simulink model "Absolute_Block_Testing"  (R2021a)
settings: Solver=VariableStepAuto  StartTime=0.0  StopTime=0.35  RelTol=1e-3
undefined symbols (not defined in the file): lambda2
libraries: dspsigops x4, dspquant2 x4
(part 1 of 2)
settings Model: Creator=hp  LastModifiedBy=hp

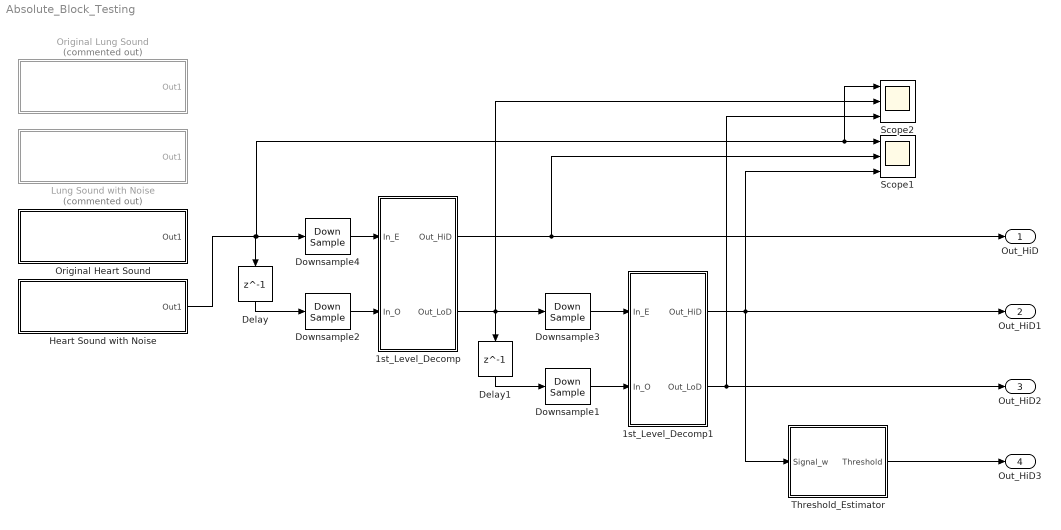
== system Absolute_Block_Testing ==
  1st_Level_Decomp : Subsystem
  1st_Level_Decomp1 : Subsystem
  Delay : Delay  DelayLength=1  SampleTime=1/44100
  Delay1 : Delay  DelayLength=1  SampleTime=1/44100
  Downsample{1..4} (4 alike) : DownSample  N=20  RateOptions=Allow multirate processing
  Heart Sound with Noise : Subsystem
  Lung Sound with Noise : Subsystem  Commented=on
  Original Heart Sound : Subsystem
  Original Lung Sound : Subsystem  Commented=on
  Scope1 : Scope  NumInputPorts=3
  Scope2 : Scope  NumInputPorts=3
  Threshold_Estimator : Subsystem
  Out_HiD : Outport  OutDataTypeStr=fixdt(1,16,12)  SampleTime=1/44100  VectorParamsAs1DForOutWhenUnconnected=off
  Out_HiD1 : Outport  Port=2  OutDataTypeStr=fixdt(1,16,12)  SampleTime=1/44100  VectorParamsAs1DForOutWhenUnconnected=off
  Out_HiD2 : Outport  Port=3  OutDataTypeStr=fixdt(1,16,12)  SampleTime=1/44100  VectorParamsAs1DForOutWhenUnconnected=off
  Out_HiD3 : Outport  Port=4  OutDataTypeStr=fixdt(1,16,12)  SampleTime=1/44100  VectorParamsAs1DForOutWhenUnconnected=off
  wires:
  Delay/1 -> Downsample2/1
  Downsample2/1 -> 1st_Level_Decomp/2(In_O)
  Downsample4/1 -> 1st_Level_Decomp/1(In_E)
  Downsample3/1 -> 1st_Level_Decomp1/1(In_E)
  Delay1/1 -> Downsample1/1
  1st_Level_Decomp/2(Out_LoD) -> Scope2/2, Delay1/1, Downsample3/1
  Downsample1/1 -> 1st_Level_Decomp1/2(In_O)
  1st_Level_Decomp1/1(Out_HiD) -> Scope1/3, Out_HiD1/1, Threshold_Estimator/1(Signal_w)
  1st_Level_Decomp/1(Out_HiD) -> Scope1/2, Out_HiD/1
  1st_Level_Decomp1/2(Out_LoD) -> Scope2/3, Out_HiD2/1
  Threshold_Estimator/1(Threshold) -> Out_HiD3/1
  Heart Sound with Noise/1(Out1) -> Delay/1, Scope1/1, Scope2/1, Downsample4/1

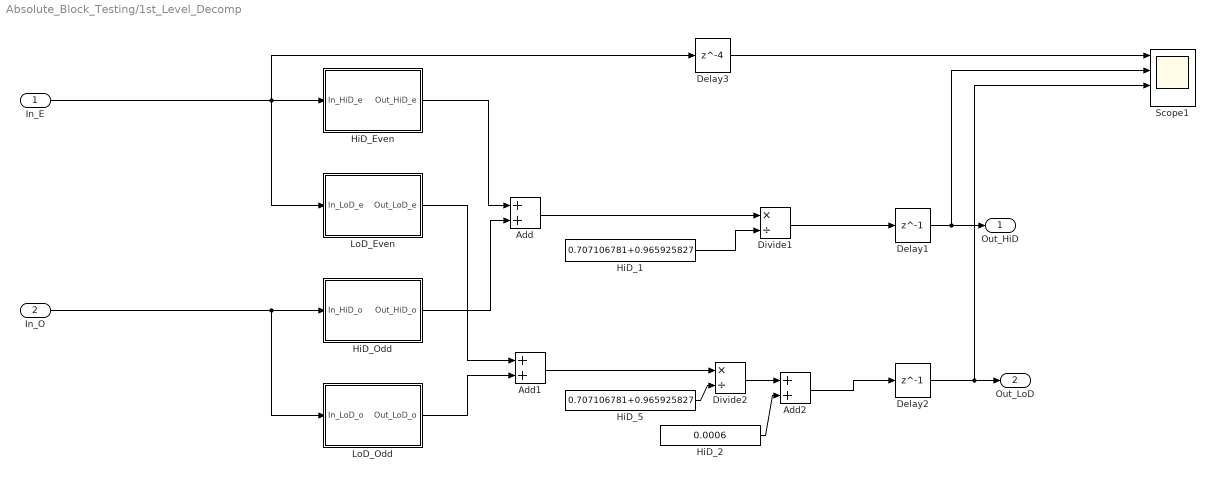
== system Absolute_Block_Testing/1st_Level_Decomp ==
  In_E : Inport  OutDataTypeStr=fixdt(1,16,12)  SampleTime=0.000022675736
  In_O : Inport  Port=2  OutDataTypeStr=fixdt(1,16,12)  SampleTime=0.000022675736
  Add : Sum  AccumDataTypeStr=fixdt(1,16,12)  OutDataTypeStr=fixdt(1,16,12)  LockScale=on
  Add1 : Sum  AccumDataTypeStr=fixdt(1,16,12)  OutDataTypeStr=fixdt(1,16,12)  LockScale=on
  Add2 : Sum  AccumDataTypeStr=fixdt(1,16,12)  OutDataTypeStr=fixdt(1,16,12)  LockScale=on
  Delay1 : Delay  DelayLength=1  SampleTime=0.000022675736
  Delay2 : Delay  DelayLength=1  SampleTime=0.000022675736
  Delay3 : Delay  DelayLength=4  SampleTime=0.000022675736
  Divide1 : Product  Inputs=*/  OutDataTypeStr=fixdt(1,16,12)
  Divide2 : Product  Inputs=*/  OutDataTypeStr=fixdt(1,16,12)
  HiD_1 : Constant  Value=0.707106781+0.965925827  OutDataTypeStr=fixdt(1,16,12)  SampleTime=1/44100
  HiD_2 : Constant  Value=0.0006  OutDataTypeStr=fixdt(1,16,12)  SampleTime=1/44100
  HiD_5 : Constant  Value=0.707106781+0.965925827  OutDataTypeStr=fixdt(1,16,12)  SampleTime=1/44100
  HiD_Even : Subsystem
  HiD_Odd : Subsystem
  LoD_Even : Subsystem
  LoD_Odd : Subsystem
  Scope1 : Scope  NumInputPorts=4
  Out_HiD : Outport  OutDataTypeStr=fixdt(1,16,12)  SampleTime=0.000022675736
  Out_LoD : Outport  Port=2  OutDataTypeStr=fixdt(1,16,12)  SampleTime=0.000022675736
  wires:
  HiD_Even/1(Out_HiD_e) -> Add/1
  HiD_Odd/1(Out_HiD_o) -> Add/2
  LoD_Even/1(Out_LoD_e) -> Add1/1
  Delay1/1 -> Scope1/2, Out_HiD/1
  Delay2/1 -> Scope1/3, Out_LoD/1
  In_E/1 -> LoD_Even/1(In_LoD_e), Delay3/1, HiD_Even/1(In_HiD_e)
  In_O/1 -> HiD_Odd/1(In_HiD_o), LoD_Odd/1(In_LoD_o)
  Add/1 -> Divide1/1
  Add1/1 -> Divide2/1
  LoD_Odd/1(Out_LoD_o) -> Add1/2
  HiD_5/1 -> Divide2/2
  HiD_1/1 -> Divide1/2
  Delay3/1 -> Scope1/1
  Divide2/1 -> Add2/1
  HiD_2/1 -> Add2/2
  Add2/1 -> Delay2/1
  Divide1/1 -> Delay1/1

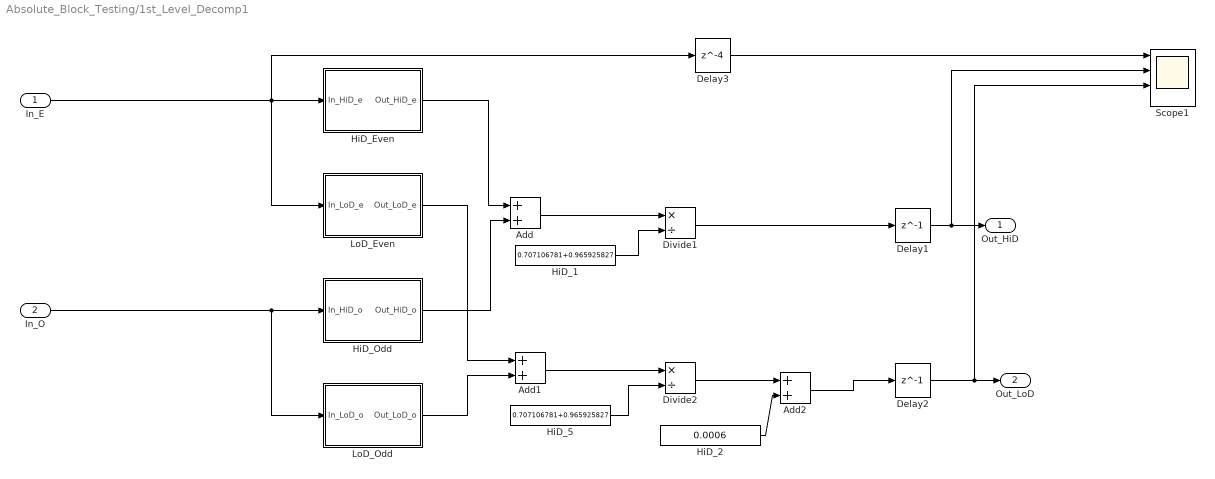
== system Absolute_Block_Testing/1st_Level_Decomp1 ==
  In_E : Inport  OutDataTypeStr=fixdt(1,16,12)  SampleTime=0.000022675736
  In_O : Inport  Port=2  OutDataTypeStr=fixdt(1,16,12)  SampleTime=0.000022675736
  Add : Sum  AccumDataTypeStr=fixdt(1,16,12)  OutDataTypeStr=fixdt(1,16,12)  LockScale=on
  Add1 : Sum  AccumDataTypeStr=fixdt(1,16,12)  OutDataTypeStr=fixdt(1,16,12)  LockScale=on
  Add2 : Sum  AccumDataTypeStr=fixdt(1,16,12)  OutDataTypeStr=fixdt(1,16,12)  LockScale=on
  Delay1 : Delay  DelayLength=1  SampleTime=0.000022675736
  Delay2 : Delay  DelayLength=1  SampleTime=0.000022675736
  Delay3 : Delay  DelayLength=4  SampleTime=0.000022675736
  Divide1 : Product  Inputs=*/  OutDataTypeStr=fixdt(1,16,12)
  Divide2 : Product  Inputs=*/  OutDataTypeStr=fixdt(1,16,12)
  HiD_1 : Constant  Value=0.707106781+0.965925827  OutDataTypeStr=fixdt(1,16,12)  SampleTime=1/44100
  HiD_2 : Constant  Value=0.0006  OutDataTypeStr=fixdt(1,16,12)  SampleTime=1/44100
  HiD_5 : Constant  Value=0.707106781+0.965925827  OutDataTypeStr=fixdt(1,16,12)  SampleTime=1/44100
  HiD_Even : Subsystem
  HiD_Odd : Subsystem
  LoD_Even : Subsystem
  LoD_Odd : Subsystem
  Scope1 : Scope  NumInputPorts=4
  Out_HiD : Outport  OutDataTypeStr=fixdt(1,16,12)  SampleTime=0.000022675736
  Out_LoD : Outport  Port=2  OutDataTypeStr=fixdt(1,16,12)  SampleTime=0.000022675736
  wires:
  HiD_Even/1(Out_HiD_e) -> Add/1
  HiD_Odd/1(Out_HiD_o) -> Add/2
  LoD_Even/1(Out_LoD_e) -> Add1/1
  Delay1/1 -> Scope1/2, Out_HiD/1
  Delay2/1 -> Scope1/3, Out_LoD/1
  In_E/1 -> LoD_Even/1(In_LoD_e), Delay3/1, HiD_Even/1(In_HiD_e)
  In_O/1 -> HiD_Odd/1(In_HiD_o), LoD_Odd/1(In_LoD_o)
  Add/1 -> Divide1/1
  Add1/1 -> Divide2/1
  LoD_Odd/1(Out_LoD_o) -> Add1/2
  HiD_5/1 -> Divide2/2
  HiD_1/1 -> Divide1/2
  Delay3/1 -> Scope1/1
  Divide2/1 -> Add2/1
  HiD_2/1 -> Add2/2
  Add2/1 -> Delay2/1
  Divide1/1 -> Delay1/1

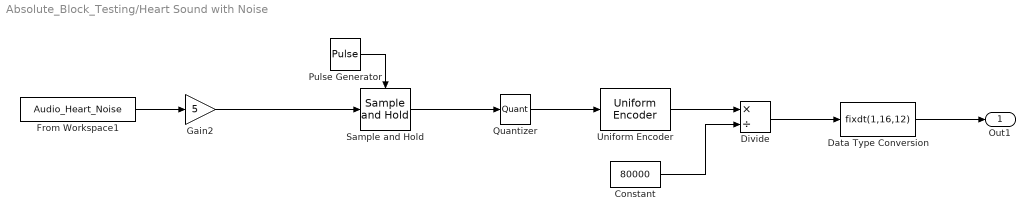
== system Absolute_Block_Testing/Heart Sound with Noise ==
  Constant : Constant  Value=80000
  Data Type Conversion : DataTypeConversion  OutDataTypeStr=fixdt(1,16,12)
  Divide : Product  Inputs=*/
  From Workspace1 : FromWorkspace  VariableName=Audio_Heart_Noise  OutDataTypeStr=double
  Gain2 : Gain  Gain=5
  Pulse Generator : DiscretePulseGenerator  PulseType=Time based  Period=0.00022675736  PulseWidth=50
  Quantizer : Quantizer  QuantizationInterval=0.1
  Sample and Hold : dspsigops/Sample and Hold  trig=Rising edge  initCond=0  latchinput=off
  Uniform Encoder : dspquant2/Uniform Encoder  peak=2  bits=8  otype=Unsigned integer
  Out1 : Outport  OutDataTypeStr=fixdt(1,16,12)  SampleTime=1/44100
  wires:
  Sample and Hold/1 -> Quantizer/1
  Uniform Encoder/1 -> Divide/1
  Divide/1 -> Data Type Conversion/1
  Quantizer/1 -> Uniform Encoder/1
  Constant/1 -> Divide/2
  From Workspace1/1 -> Gain2/1
  Pulse Generator/1 -> Sample and Hold/Trigger
  Gain2/1 -> Sample and Hold/1
  Data Type Conversion/1 -> Out1/1

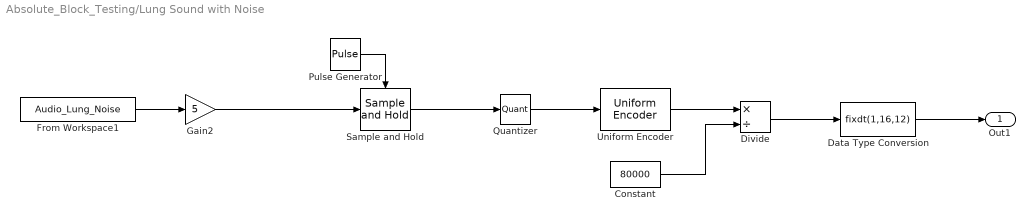
== system Absolute_Block_Testing/Lung Sound with Noise ==
  Constant : Constant  Value=80000
  Data Type Conversion : DataTypeConversion  OutDataTypeStr=fixdt(1,16,12)
  Divide : Product  Inputs=*/
  From Workspace1 : FromWorkspace  VariableName=Audio_Lung_Noise  OutDataTypeStr=double
  Gain2 : Gain  Gain=5
  Pulse Generator : DiscretePulseGenerator  PulseType=Time based  Period=0.00022675736  PulseWidth=50
  Quantizer : Quantizer  QuantizationInterval=0.1
  Sample and Hold : dspsigops/Sample and Hold  trig=Rising edge  initCond=0  latchinput=off
  Uniform Encoder : dspquant2/Uniform Encoder  peak=2  bits=8  otype=Unsigned integer
  Out1 : Outport  OutDataTypeStr=fixdt(1,16,12)  SampleTime=1/44100
  wires:
  Sample and Hold/1 -> Quantizer/1
  Uniform Encoder/1 -> Divide/1
  Divide/1 -> Data Type Conversion/1
  Quantizer/1 -> Uniform Encoder/1
  Constant/1 -> Divide/2
  From Workspace1/1 -> Gain2/1
  Pulse Generator/1 -> Sample and Hold/Trigger
  Gain2/1 -> Sample and Hold/1
  Data Type Conversion/1 -> Out1/1

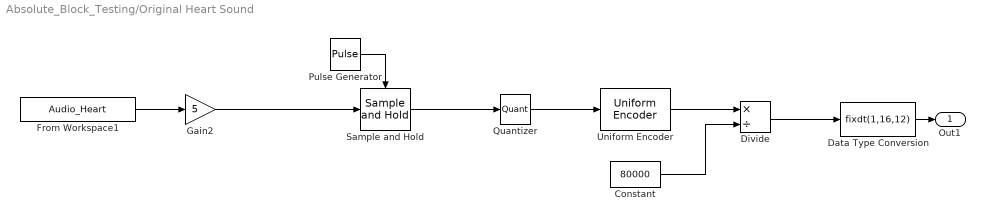
== system Absolute_Block_Testing/Original Heart Sound ==
  Constant : Constant  Value=80000
  Data Type Conversion : DataTypeConversion  OutDataTypeStr=fixdt(1,16,12)
  Divide : Product  Inputs=*/
  From Workspace1 : FromWorkspace  VariableName=Audio_Heart  OutDataTypeStr=double
  Gain2 : Gain  Gain=5
  Pulse Generator : DiscretePulseGenerator  PulseType=Time based  Period=0.00022675736  PulseWidth=50
  Quantizer : Quantizer  QuantizationInterval=0.1
  Sample and Hold : dspsigops/Sample and Hold  trig=Rising edge  initCond=0  latchinput=off
  Uniform Encoder : dspquant2/Uniform Encoder  peak=2  bits=8  otype=Unsigned integer
  Out1 : Outport  OutDataTypeStr=fixdt(1,16,12)  SampleTime=1/44100
  wires:
  Sample and Hold/1 -> Quantizer/1
  Uniform Encoder/1 -> Divide/1
  Divide/1 -> Data Type Conversion/1
  Quantizer/1 -> Uniform Encoder/1
  Constant/1 -> Divide/2
  From Workspace1/1 -> Gain2/1
  Pulse Generator/1 -> Sample and Hold/Trigger
  Gain2/1 -> Sample and Hold/1
  Data Type Conversion/1 -> Out1/1

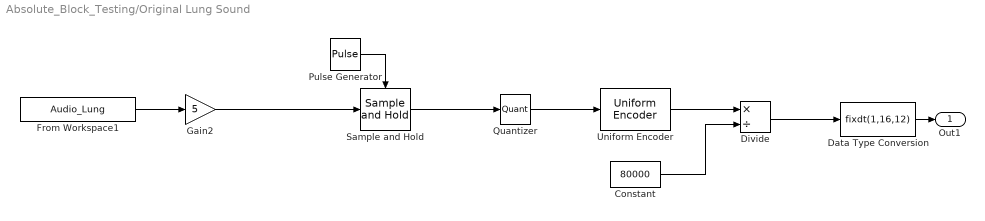
== system Absolute_Block_Testing/Original Lung Sound ==
  Constant : Constant  Value=80000
  Data Type Conversion : DataTypeConversion  OutDataTypeStr=fixdt(1,16,12)
  Divide : Product  Inputs=*/
  From Workspace1 : FromWorkspace  VariableName=Audio_Lung  OutDataTypeStr=double
  Gain2 : Gain  Gain=5
  Pulse Generator : DiscretePulseGenerator  PulseType=Time based  Period=0.00022675736  PulseWidth=50
  Quantizer : Quantizer  QuantizationInterval=0.1
  Sample and Hold : dspsigops/Sample and Hold  trig=Rising edge  initCond=0  latchinput=off
  Uniform Encoder : dspquant2/Uniform Encoder  peak=2  bits=8  otype=Unsigned integer
  Out1 : Outport  OutDataTypeStr=fixdt(1,16,12)
  wires:
  Sample and Hold/1 -> Quantizer/1
  Uniform Encoder/1 -> Divide/1
  Divide/1 -> Data Type Conversion/1
  Quantizer/1 -> Uniform Encoder/1
  Constant/1 -> Divide/2
  From Workspace1/1 -> Gain2/1
  Pulse Generator/1 -> Sample and Hold/Trigger
  Gain2/1 -> Sample and Hold/1
  Data Type Conversion/1 -> Out1/1

== system Absolute_Block_Testing/Threshold_Estimator ==
  Signal_w : Inport  OutDataTypeStr=fixdt(1,16,12)  SampleTime=0.000022675736
  Absolute Signal : Scope
  Absolute_Value1 : Subsystem
  Detailed SIgnal : Scope
  Length : Constant  Value=lambda2  OutDataTypeStr=fixdt(1,16,12)  SampleTime=0.000022675736
  Median2 : Subsystem
  Multiply : Product  OutDataTypeStr=fixdt(1,16,12)  LockScale=on
  Scope3 : Scope  NumInputPorts=2
  Threshold : Outport  OutDataTypeStr=fixdt(1,16,12)  SampleTime=0.000022675736  VectorParamsAs1DForOutWhenUnconnected=off
  wires:
  Length/1 -> Multiply/2
  Median2/1(Median) -> Multiply/1
  Absolute_Value1/1(Out_Abs) -> Absolute Signal/1, Scope3/2, Median2/1(Signal_w3)
  Signal_w/1 -> Detailed SIgnal/1, Scope3/1, Absolute_Value1/1(Signal_w4)
  Multiply/1 -> Threshold/1

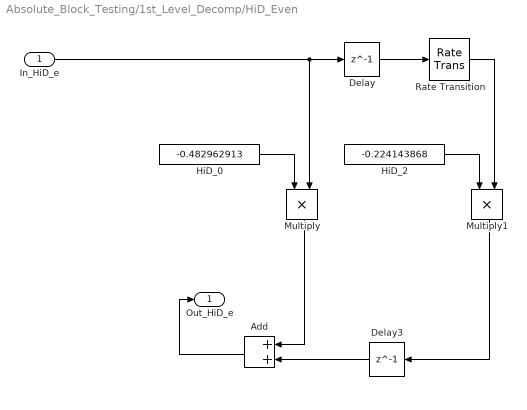
== system Absolute_Block_Testing/1st_Level_Decomp/HiD_Even ==
  In_HiD_e : Inport  OutDataTypeStr=fixdt(1,16,12)  SampleTime=0.000022675736
  Add : Sum  AccumDataTypeStr=fixdt(1,16,12)  OutDataTypeStr=fixdt(1,16,12)  LockScale=on
  Delay : Delay  DelayLength=1  SampleTime=0.000022675736
  Delay3 : Delay  DelayLength=1  SampleTime=0.000022675736
  HiD_0 : Constant  Value=-0.482962913  OutDataTypeStr=fixdt(1,16,12)  SampleTime=0.000022675736
  HiD_2 : Constant  Value=-0.224143868  OutDataTypeStr=fixdt(1,16,12)  SampleTime=0.000022675736
  Multiply : Product  OutDataTypeStr=fixdt(1,16,12)  LockScale=on
  Multiply1 : Product  OutDataTypeStr=fixdt(1,16,12)  LockScale=on
  Rate Transition : RateTransition  OutPortSampleTime=0.000022675736
  Out_HiD_e : Outport  OutDataTypeStr=fixdt(1,16,12)  SampleTime=0.000022675736  VectorParamsAs1DForOutWhenUnconnected=off
  wires:
  Delay/1 -> Rate Transition/1
  Delay3/1 -> Add/2
  Multiply1/1 -> Delay3/1
  Multiply/1 -> Add/1
  HiD_0/1 -> Multiply/1
  HiD_2/1 -> Multiply1/1
  Add/1 -> Out_HiD_e/1
  In_HiD_e/1 -> Multiply/2, Delay/1
  Rate Transition/1 -> Multiply1/2

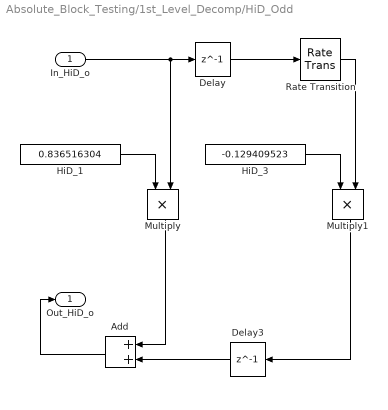
== system Absolute_Block_Testing/1st_Level_Decomp/HiD_Odd ==
  In_HiD_o : Inport  OutDataTypeStr=fixdt(1,16,12)  SampleTime=0.000022675736
  Add : Sum  AccumDataTypeStr=fixdt(1,16,12)  OutDataTypeStr=fixdt(1,16,12)  LockScale=on
  Delay : Delay  DelayLength=1  SampleTime=0.000022675736
  Delay3 : Delay  DelayLength=1  SampleTime=0.000022675736
  HiD_1 : Constant  Value=0.836516304  OutDataTypeStr=fixdt(1,16,12)  SampleTime=0
  HiD_3 : Constant  Value=-0.129409523  OutDataTypeStr=fixdt(1,16,12)  SampleTime=0
  Multiply : Product  OutDataTypeStr=fixdt(1,16,12)  LockScale=on
  Multiply1 : Product  OutDataTypeStr=fixdt(1,16,12)  LockScale=on
  Rate Transition : RateTransition  OutPortSampleTime=0.000022675736
  Out_HiD_o : Outport  OutDataTypeStr=fixdt(1,16,12)  SampleTime=0.000022675736  VectorParamsAs1DForOutWhenUnconnected=off
  wires:
  Delay/1 -> Rate Transition/1
  Delay3/1 -> Add/2
  Multiply1/1 -> Delay3/1
  Multiply/1 -> Add/1
  HiD_1/1 -> Multiply/1
  HiD_3/1 -> Multiply1/1
  Add/1 -> Out_HiD_o/1
  In_HiD_o/1 -> Delay/1, Multiply/2
  Rate Transition/1 -> Multiply1/2

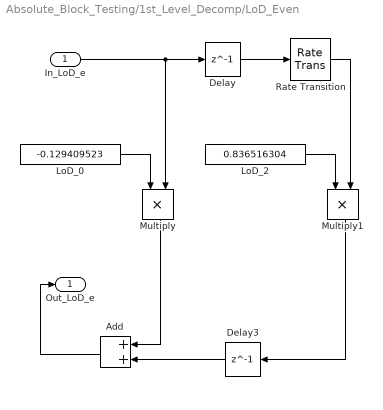
== system Absolute_Block_Testing/1st_Level_Decomp/LoD_Even ==
  In_LoD_e : Inport  OutDataTypeStr=fixdt(1,16,12)  SampleTime=0.000022675736
  Add : Sum  AccumDataTypeStr=fixdt(1,16,12)  OutDataTypeStr=fixdt(1,16,12)  LockScale=on
  Delay : Delay  DelayLength=1  SampleTime=0.000022675736
  Delay3 : Delay  DelayLength=1  SampleTime=0.000022675736
  LoD_0 : Constant  Value=-0.129409523  OutDataTypeStr=fixdt(1,16,12)  SampleTime=0
  LoD_2 : Constant  Value=0.836516304  OutDataTypeStr=fixdt(1,16,12)  SampleTime=0
  Multiply : Product  OutDataTypeStr=fixdt(1,16,12)  LockScale=on
  Multiply1 : Product  OutDataTypeStr=fixdt(1,16,12)  LockScale=on
  Rate Transition : RateTransition  OutPortSampleTime=0.000022675736
  Out_LoD_e : Outport  OutDataTypeStr=fixdt(1,16,12)  SampleTime=0.000022675736  VectorParamsAs1DForOutWhenUnconnected=off
  wires:
  Delay/1 -> Rate Transition/1
  Delay3/1 -> Add/2
  Multiply1/1 -> Delay3/1
  Multiply/1 -> Add/1
  LoD_0/1 -> Multiply/1
  LoD_2/1 -> Multiply1/1
  Add/1 -> Out_LoD_e/1
  In_LoD_e/1 -> Delay/1, Multiply/2
  Rate Transition/1 -> Multiply1/2

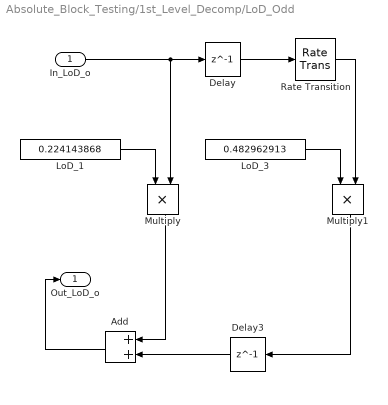
== system Absolute_Block_Testing/1st_Level_Decomp/LoD_Odd ==
  In_LoD_o : Inport  OutDataTypeStr=fixdt(1,16,12)  SampleTime=0.000022675736
  Add : Sum  AccumDataTypeStr=fixdt(1,16,12)  OutDataTypeStr=fixdt(1,16,12)  LockScale=on
  Delay : Delay  DelayLength=1  SampleTime=0.000022675736
  Delay3 : Delay  DelayLength=1  SampleTime=0.000022675736
  LoD_1 : Constant  Value=0.224143868  OutDataTypeStr=fixdt(1,16,12)  SampleTime=0
  LoD_3 : Constant  Value=0.482962913  OutDataTypeStr=fixdt(1,16,12)  SampleTime=0
  Multiply : Product  OutDataTypeStr=fixdt(1,16,12)  LockScale=on
  Multiply1 : Product  OutDataTypeStr=fixdt(1,16,12)  LockScale=on
  Rate Transition : RateTransition  OutPortSampleTime=0.000022675736
  Out_LoD_o : Outport  OutDataTypeStr=fixdt(1,16,12)  SampleTime=0.000022675736  VectorParamsAs1DForOutWhenUnconnected=off
  wires:
  Delay/1 -> Rate Transition/1
  Delay3/1 -> Add/2
  Multiply1/1 -> Delay3/1
  Multiply/1 -> Add/1
  LoD_1/1 -> Multiply/1
  LoD_3/1 -> Multiply1/1
  Add/1 -> Out_LoD_o/1
  In_LoD_o/1 -> Delay/1, Multiply/2
  Rate Transition/1 -> Multiply1/2

== system Absolute_Block_Testing/1st_Level_Decomp1/HiD_Even ==
  In_HiD_e : Inport  OutDataTypeStr=fixdt(1,16,12)  SampleTime=0.000022675736
  Add : Sum  AccumDataTypeStr=fixdt(1,16,12)  OutDataTypeStr=fixdt(1,16,12)  LockScale=on
  Delay : Delay  DelayLength=1  SampleTime=0.000022675736
  Delay3 : Delay  DelayLength=1  SampleTime=0.000022675736
  HiD_0 : Constant  Value=-0.482962913  OutDataTypeStr=fixdt(1,16,12)  SampleTime=0.000022675736
  HiD_2 : Constant  Value=-0.224143868  OutDataTypeStr=fixdt(1,16,12)  SampleTime=0.000022675736
  Multiply : Product  OutDataTypeStr=fixdt(1,16,12)  LockScale=on
  Multiply1 : Product  OutDataTypeStr=fixdt(1,16,12)  LockScale=on
  Rate Transition : RateTransition  OutPortSampleTime=0.000022675736
  Out_HiD_e : Outport  OutDataTypeStr=fixdt(1,16,12)  SampleTime=0.000022675736  VectorParamsAs1DForOutWhenUnconnected=off
  wires:
  Delay/1 -> Rate Transition/1
  Delay3/1 -> Add/2
  Multiply1/1 -> Delay3/1
  Multiply/1 -> Add/1
  HiD_0/1 -> Multiply/1
  HiD_2/1 -> Multiply1/1
  Add/1 -> Out_HiD_e/1
  In_HiD_e/1 -> Multiply/2, Delay/1
  Rate Transition/1 -> Multiply1/2

== system Absolute_Block_Testing/1st_Level_Decomp1/HiD_Odd ==
  In_HiD_o : Inport  OutDataTypeStr=fixdt(1,16,12)  SampleTime=0.000022675736
  Add : Sum  AccumDataTypeStr=fixdt(1,16,12)  OutDataTypeStr=fixdt(1,16,12)  LockScale=on
  Delay : Delay  DelayLength=1  SampleTime=0.000022675736
  Delay3 : Delay  DelayLength=1  SampleTime=0.000022675736
  HiD_1 : Constant  Value=0.836516304  OutDataTypeStr=fixdt(1,16,12)  SampleTime=0
  HiD_3 : Constant  Value=-0.129409523  OutDataTypeStr=fixdt(1,16,12)  SampleTime=0
  Multiply : Product  OutDataTypeStr=fixdt(1,16,12)  LockScale=on
  Multiply1 : Product  OutDataTypeStr=fixdt(1,16,12)  LockScale=on
  Rate Transition : RateTransition  OutPortSampleTime=0.000022675736
  Out_HiD_o : Outport  OutDataTypeStr=fixdt(1,16,12)  SampleTime=0.000022675736  VectorParamsAs1DForOutWhenUnconnected=off
  wires:
  Delay/1 -> Rate Transition/1
  Delay3/1 -> Add/2
  Multiply1/1 -> Delay3/1
  Multiply/1 -> Add/1
  HiD_1/1 -> Multiply/1
  HiD_3/1 -> Multiply1/1
  Add/1 -> Out_HiD_o/1
  In_HiD_o/1 -> Delay/1, Multiply/2
  Rate Transition/1 -> Multiply1/2

== system Absolute_Block_Testing/1st_Level_Decomp1/LoD_Even ==
  In_LoD_e : Inport  OutDataTypeStr=fixdt(1,16,12)  SampleTime=0.000022675736
  Add : Sum  AccumDataTypeStr=fixdt(1,16,12)  OutDataTypeStr=fixdt(1,16,12)  LockScale=on
  Delay : Delay  DelayLength=1  SampleTime=0.000022675736
  Delay3 : Delay  DelayLength=1  SampleTime=0.000022675736
  LoD_0 : Constant  Value=-0.129409523  OutDataTypeStr=fixdt(1,16,12)  SampleTime=0
  LoD_2 : Constant  Value=0.836516304  OutDataTypeStr=fixdt(1,16,12)  SampleTime=0
  Multiply : Product  OutDataTypeStr=fixdt(1,16,12)  LockScale=on
  Multiply1 : Product  OutDataTypeStr=fixdt(1,16,12)  LockScale=on
  Rate Transition : RateTransition  OutPortSampleTime=0.000022675736
  Out_LoD_e : Outport  OutDataTypeStr=fixdt(1,16,12)  SampleTime=0.000022675736  VectorParamsAs1DForOutWhenUnconnected=off
  wires:
  Delay/1 -> Rate Transition/1
  Delay3/1 -> Add/2
  Multiply1/1 -> Delay3/1
  Multiply/1 -> Add/1
  LoD_0/1 -> Multiply/1
  LoD_2/1 -> Multiply1/1
  Add/1 -> Out_LoD_e/1
  In_LoD_e/1 -> Delay/1, Multiply/2
  Rate Transition/1 -> Multiply1/2

== system Absolute_Block_Testing/1st_Level_Decomp1/LoD_Odd ==
  In_LoD_o : Inport  OutDataTypeStr=fixdt(1,16,12)  SampleTime=0.000022675736
  Add : Sum  AccumDataTypeStr=fixdt(1,16,12)  OutDataTypeStr=fixdt(1,16,12)  LockScale=on
  Delay : Delay  DelayLength=1  SampleTime=0.000022675736
  Delay3 : Delay  DelayLength=1  SampleTime=0.000022675736
  LoD_1 : Constant  Value=0.224143868  OutDataTypeStr=fixdt(1,16,12)  SampleTime=0
  LoD_3 : Constant  Value=0.482962913  OutDataTypeStr=fixdt(1,16,12)  SampleTime=0
  Multiply : Product  OutDataTypeStr=fixdt(1,16,12)  LockScale=on
  Multiply1 : Product  OutDataTypeStr=fixdt(1,16,12)  LockScale=on
  Rate Transition : RateTransition  OutPortSampleTime=0.000022675736
  Out_LoD_o : Outport  OutDataTypeStr=fixdt(1,16,12)  SampleTime=0.000022675736  VectorParamsAs1DForOutWhenUnconnected=off
  wires:
  Delay/1 -> Rate Transition/1
  Delay3/1 -> Add/2
  Multiply1/1 -> Delay3/1
  Multiply/1 -> Add/1
  LoD_1/1 -> Multiply/1
  LoD_3/1 -> Multiply1/1
  Add/1 -> Out_LoD_o/1
  In_LoD_o/1 -> Delay/1, Multiply/2
  Rate Transition/1 -> Multiply1/2

== system Absolute_Block_Testing/Threshold_Estimator/Absolute_Value1 ==
  Signal_w4 : Inport  OutDataTypeStr=fixdt(1,16,12)  SampleTime=0.000022675736
  Absolute_Switch : Switch  Threshold=1  OutDataTypeStr=fixdt(1,16,12)
  Constant295 : Constant  Value=0  OutDataTypeStr=fixdt(1,16,12)  SampleTime=0.000022675736
  Gain2 : Gain  Gain=-1  ParamDataTypeStr=fixdt(1,16,0)  OutMin=-1  OutMax=-0.99  OutDataTypeStr=fixdt(1,16,12)
  Relational Operator2 : RelationalOperator  Operator=<  OutDataTypeStr=fixdt(1,16,12)  RndMeth=Simplest
  Out_Abs : Outport  OutDataTypeStr=fixdt(1,16,12)  SampleTime=0.000022675736  VectorParamsAs1DForOutWhenUnconnected=off
  wires:
  Absolute_Switch/1 -> Out_Abs/1
  Relational Operator2/1 -> Absolute_Switch/2
  Gain2/1 -> Absolute_Switch/1
  Signal_w4/1 -> Absolute_Switch/3, Relational Operator2/1, Gain2/1
  Constant295/1 -> Relational Operator2/2

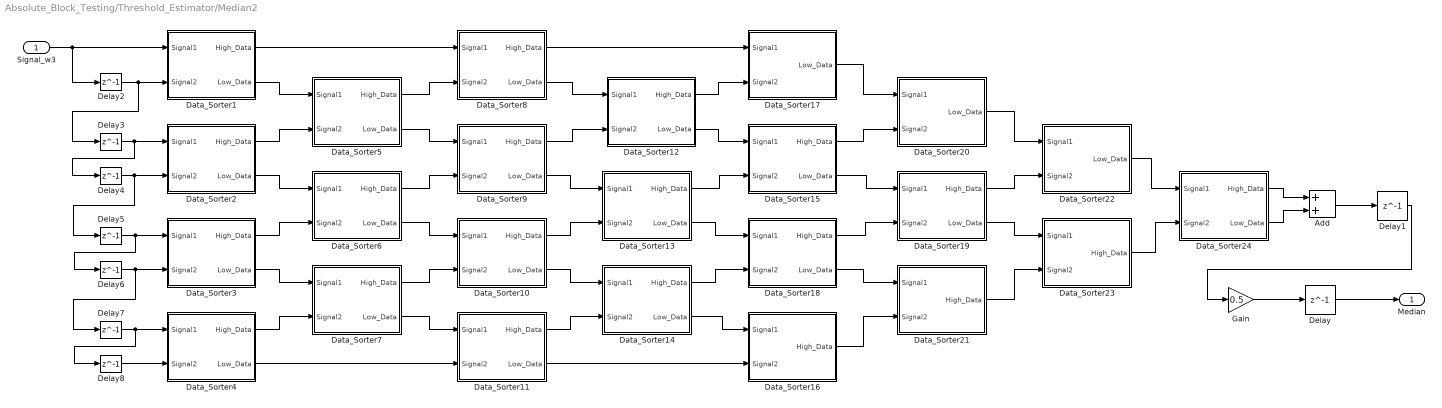
== system Absolute_Block_Testing/Threshold_Estimator/Median2 ==
  Signal_w3 : Inport  OutDataTypeStr=fixdt(1,16,12)  SampleTime=0.000022675736
  Add : Sum  AccumDataTypeStr=fixdt(1,16,12)  OutDataTypeStr=fixdt(1,16,12)  LockScale=on
  Data_Sorter1 : Subsystem
  Data_Sorter10 : Subsystem
  Data_Sorter11 : Subsystem
  Data_Sorter12 : Subsystem
  Data_Sorter13 : Subsystem
  Data_Sorter14 : Subsystem
  Data_Sorter15 : Subsystem
  Data_Sorter16 : Subsystem
  Data_Sorter17 : Subsystem
  Data_Sorter18 : Subsystem
  Data_Sorter19 : Subsystem
  Data_Sorter2 : Subsystem
  Data_Sorter20 : Subsystem
  Data_Sorter21 : Subsystem
  Data_Sorter22 : Subsystem
  Data_Sorter23 : Subsystem
  Data_Sorter24 : Subsystem
  Data_Sorter3 : Subsystem
  Data_Sorter4 : Subsystem
  Data_Sorter5 : Subsystem
  Data_Sorter6 : Subsystem
  Data_Sorter7 : Subsystem
  Data_Sorter8 : Subsystem
  Data_Sorter9 : Subsystem
  Delay{,1..8} (9 alike) : Delay  DelayLength=1  SampleTime=0.000022675736
  Gain : Gain  Gain=0.5  ParamDataTypeStr=fixdt(1,16,12)  OutMin=0.499  OutMax=0.5  OutDataTypeStr=fixdt(1,16,12)
  Median : Outport  OutDataTypeStr=fixdt(1,16,12)  SampleTime=0.000022675736  VectorParamsAs1DForOutWhenUnconnected=off
  wires:
  Data_Sorter4/1(High_Data) -> Data_Sorter7/2(Signal2)
  Delay3/1 -> Data_Sorter2/1(Signal1), Delay4/1
  Signal_w3/1 -> Data_Sorter1/1(Signal1), Delay2/1
  Data_Sorter10/1(High_Data) -> Data_Sorter13/2(Signal2)
  Data_Sorter23/1(High_Data) -> Data_Sorter24/2(Signal2)
  Data_Sorter12/2(Low_Data) -> Data_Sorter15/1(Signal1)
  Delay2/1 -> Delay3/1, Data_Sorter1/2(Signal2)
  Data_Sorter5/1(High_Data) -> Data_Sorter8/2(Signal2)
  Delay/1 -> Median/1
  Data_Sorter17/1(Low_Data) -> Data_Sorter20/1(Signal1)
  Add/1 -> Delay1/1
  Data_Sorter7/2(Low_Data) -> Data_Sorter11/1(Signal1)
  Data_Sorter24/1(High_Data) -> Add/1
  Data_Sorter1/2(Low_Data) -> Data_Sorter5/1(Signal1)
  Data_Sorter3/1(High_Data) -> Data_Sorter6/2(Signal2)
  Data_Sorter22/1(Low_Data) -> Data_Sorter24/1(Signal1)
  Data_Sorter2/1(High_Data) -> Data_Sorter5/2(Signal2)
  Data_Sorter10/2(Low_Data) -> Data_Sorter14/1(Signal1)
  Delay1/1 -> Gain/1
  Data_Sorter18/2(Low_Data) -> Data_Sorter21/1(Signal1)
  Data_Sorter21/1(High_Data) -> Data_Sorter23/2(Signal2)
  Data_Sorter7/1(High_Data) -> Data_Sorter10/2(Signal2)
  Delay4/1 -> Data_Sorter2/2(Signal2), Delay5/1
  Data_Sorter15/1(High_Data) -> Data_Sorter20/2(Signal2)
  Data_Sorter19/1(High_Data) -> Data_Sorter22/2(Signal2)
  Data_Sorter15/2(Low_Data) -> Data_Sorter19/1(Signal1)
  Data_Sorter3/2(Low_Data) -> Data_Sorter7/1(Signal1)
  Data_Sorter2/2(Low_Data) -> Data_Sorter6/1(Signal1)
  Data_Sorter6/2(Low_Data) -> Data_Sorter10/1(Signal1)
  Data_Sorter20/1(Low_Data) -> Data_Sorter22/1(Signal1)
  Data_Sorter12/1(High_Data) -> Data_Sorter17/2(Signal2)
  Data_Sorter5/2(Low_Data) -> Data_Sorter9/1(Signal1)
  Data_Sorter24/2(Low_Data) -> Add/2
  Data_Sorter18/1(High_Data) -> Data_Sorter19/2(Signal2)
  Data_Sorter13/1(High_Data) -> Data_Sorter15/2(Signal2)
  Data_Sorter11/1(High_Data) -> Data_Sorter14/2(Signal2)
  Delay8/1 -> Data_Sorter4/2(Signal2)
  Data_Sorter8/2(Low_Data) -> Data_Sorter12/1(Signal1)
  Delay6/1 -> Data_Sorter3/2(Signal2), Delay7/1
  Data_Sorter9/2(Low_Data) -> Data_Sorter13/1(Signal1)
  Data_Sorter4/2(Low_Data) -> Data_Sorter11/2(Signal2)
  Data_Sorter9/1(High_Data) -> Data_Sorter12/2(Signal2)
  Data_Sorter14/2(Low_Data) -> Data_Sorter16/1(Signal1)
  Delay5/1 -> Data_Sorter3/1(Signal1), Delay6/1
  Delay7/1 -> Data_Sorter4/1(Signal1), Delay8/1
  Data_Sorter1/1(High_Data) -> Data_Sorter8/1(Signal1)
  Data_Sorter8/1(High_Data) -> Data_Sorter17/1(Signal1)
  Data_Sorter14/1(High_Data) -> Data_Sorter18/2(Signal2)
  Data_Sorter6/1(High_Data) -> Data_Sorter9/2(Signal2)
  Data_Sorter19/2(Low_Data) -> Data_Sorter23/1(Signal1)
  Data_Sorter11/2(Low_Data) -> Data_Sorter16/2(Signal2)
  Data_Sorter13/2(Low_Data) -> Data_Sorter18/1(Signal1)
  Gain/1 -> Delay/1
  Data_Sorter16/1(High_Data) -> Data_Sorter21/2(Signal2)

== system Absolute_Block_Testing/Threshold_Estimator/Median2/Data_Sorter1 ==
  Signal1 : Inport  OutDataTypeStr=fixdt(1,16,12)  SampleTime=0.000022675736
  Signal2 : Inport  Port=2  OutDataTypeStr=fixdt(1,16,12)  SampleTime=0.000022675736
  Data_Sorter_Switch : Switch  OutDataTypeStr=fixdt(1,16,12)
  Data_Sorter_Switch1 : Switch  Threshold=1  OutDataTypeStr=fixdt(1,16,12)
  Delay1 : Delay  DelayLength=1  SampleTime=0.000022675736
  Delay2 : Delay  DelayLength=1  SampleTime=0.000022675736
  Relational Operator2 : RelationalOperator  Operator=<  OutDataTypeStr=fixdt(1,16,12)  RndMeth=Simplest
  High_Data : Outport  OutDataTypeStr=fixdt(1,16,12)  SampleTime=0.000022675736  VectorParamsAs1DForOutWhenUnconnected=off
  Low_Data : Outport  Port=2  OutDataTypeStr=fixdt(1,16,12)  SampleTime=0.000022675736  VectorParamsAs1DForOutWhenUnconnected=off
  wires:
  Signal1/1 -> Data_Sorter_Switch/3, Data_Sorter_Switch/1, Relational Operator2/1
  Relational Operator2/1 -> Data_Sorter_Switch1/2, Data_Sorter_Switch/2
  Signal2/1 -> Data_Sorter_Switch1/1, Data_Sorter_Switch1/3, Relational Operator2/2
  Data_Sorter_Switch1/1 -> Delay2/1
  Delay2/1 -> Low_Data/1
  Data_Sorter_Switch/1 -> Delay1/1
  Delay1/1 -> High_Data/1

== system Absolute_Block_Testing/Threshold_Estimator/Median2/Data_Sorter10 ==
  Signal1 : Inport  OutDataTypeStr=fixdt(1,16,12)  SampleTime=0.000022675736
  Signal2 : Inport  Port=2  OutDataTypeStr=fixdt(1,16,12)  SampleTime=0.000022675736
  Data_Sorter_Switch : Switch  OutDataTypeStr=fixdt(1,16,12)
  Data_Sorter_Switch1 : Switch  Threshold=1  OutDataTypeStr=fixdt(1,16,12)
  Delay1 : Delay  DelayLength=1  SampleTime=0.000022675736
  Delay2 : Delay  DelayLength=1  SampleTime=0.000022675736
  Relational Operator2 : RelationalOperator  Operator=<  OutDataTypeStr=fixdt(1,16,12)  RndMeth=Simplest
  High_Data : Outport  OutDataTypeStr=fixdt(1,16,12)  SampleTime=0.000022675736  VectorParamsAs1DForOutWhenUnconnected=off
  Low_Data : Outport  Port=2  OutDataTypeStr=fixdt(1,16,12)  SampleTime=0.000022675736  VectorParamsAs1DForOutWhenUnconnected=off
  wires:
  Signal1/1 -> Data_Sorter_Switch/3, Data_Sorter_Switch/1, Relational Operator2/1
  Relational Operator2/1 -> Data_Sorter_Switch1/2, Data_Sorter_Switch/2
  Signal2/1 -> Data_Sorter_Switch1/1, Data_Sorter_Switch1/3, Relational Operator2/2
  Data_Sorter_Switch1/1 -> Delay2/1
  Delay2/1 -> Low_Data/1
  Data_Sorter_Switch/1 -> Delay1/1
  Delay1/1 -> High_Data/1

== system Absolute_Block_Testing/Threshold_Estimator/Median2/Data_Sorter11 ==
  Signal1 : Inport  OutDataTypeStr=fixdt(1,16,12)  SampleTime=0.000022675736
  Signal2 : Inport  Port=2  OutDataTypeStr=fixdt(1,16,12)  SampleTime=0.000022675736
  Data_Sorter_Switch : Switch  OutDataTypeStr=fixdt(1,16,12)
  Data_Sorter_Switch1 : Switch  Threshold=1  OutDataTypeStr=fixdt(1,16,12)
  Delay1 : Delay  DelayLength=1  SampleTime=0.000022675736
  Delay2 : Delay  DelayLength=1  SampleTime=0.000022675736
  Relational Operator2 : RelationalOperator  Operator=<  OutDataTypeStr=fixdt(1,16,12)  RndMeth=Simplest
  High_Data : Outport  OutDataTypeStr=fixdt(1,16,12)  SampleTime=0.000022675736  VectorParamsAs1DForOutWhenUnconnected=off
  Low_Data : Outport  Port=2  OutDataTypeStr=fixdt(1,16,12)  SampleTime=0.000022675736  VectorParamsAs1DForOutWhenUnconnected=off
  wires:
  Signal1/1 -> Data_Sorter_Switch/3, Data_Sorter_Switch/1, Relational Operator2/1
  Relational Operator2/1 -> Data_Sorter_Switch1/2, Data_Sorter_Switch/2
  Signal2/1 -> Data_Sorter_Switch1/1, Data_Sorter_Switch1/3, Relational Operator2/2
  Data_Sorter_Switch1/1 -> Delay2/1
  Delay2/1 -> Low_Data/1
  Data_Sorter_Switch/1 -> Delay1/1
  Delay1/1 -> High_Data/1

== system Absolute_Block_Testing/Threshold_Estimator/Median2/Data_Sorter12 ==
  Signal1 : Inport  OutDataTypeStr=fixdt(1,16,12)  SampleTime=0.000022675736
  Signal2 : Inport  Port=2  OutDataTypeStr=fixdt(1,16,12)  SampleTime=0.000022675736
  Data_Sorter_Switch : Switch  OutDataTypeStr=fixdt(1,16,12)
  Data_Sorter_Switch1 : Switch  Threshold=1  OutDataTypeStr=fixdt(1,16,12)
  Delay1 : Delay  DelayLength=1  SampleTime=0.000022675736
  Delay2 : Delay  DelayLength=1  SampleTime=0.000022675736
  Relational Operator2 : RelationalOperator  Operator=<  OutDataTypeStr=fixdt(1,16,12)  RndMeth=Simplest
  High_Data : Outport  OutDataTypeStr=fixdt(1,16,12)  SampleTime=0.000022675736  VectorParamsAs1DForOutWhenUnconnected=off
  Low_Data : Outport  Port=2  OutDataTypeStr=fixdt(1,16,12)  SampleTime=0.000022675736  VectorParamsAs1DForOutWhenUnconnected=off
  wires:
  Signal1/1 -> Data_Sorter_Switch/3, Data_Sorter_Switch/1, Relational Operator2/1
  Relational Operator2/1 -> Data_Sorter_Switch1/2, Data_Sorter_Switch/2
  Signal2/1 -> Data_Sorter_Switch1/1, Data_Sorter_Switch1/3, Relational Operator2/2
  Data_Sorter_Switch1/1 -> Delay2/1
  Delay2/1 -> Low_Data/1
  Data_Sorter_Switch/1 -> Delay1/1
  Delay1/1 -> High_Data/1

== system Absolute_Block_Testing/Threshold_Estimator/Median2/Data_Sorter13 ==
  Signal1 : Inport  OutDataTypeStr=fixdt(1,16,12)  SampleTime=0.000022675736
  Signal2 : Inport  Port=2  OutDataTypeStr=fixdt(1,16,12)  SampleTime=0.000022675736
  Data_Sorter_Switch : Switch  OutDataTypeStr=fixdt(1,16,12)
  Data_Sorter_Switch1 : Switch  Threshold=1  OutDataTypeStr=fixdt(1,16,12)
  Delay1 : Delay  DelayLength=1  SampleTime=0.000022675736
  Delay2 : Delay  DelayLength=1  SampleTime=0.000022675736
  Relational Operator2 : RelationalOperator  Operator=<  OutDataTypeStr=fixdt(1,16,12)  RndMeth=Simplest
  High_Data : Outport  OutDataTypeStr=fixdt(1,16,12)  SampleTime=0.000022675736  VectorParamsAs1DForOutWhenUnconnected=off
  Low_Data : Outport  Port=2  OutDataTypeStr=fixdt(1,16,12)  SampleTime=0.000022675736  VectorParamsAs1DForOutWhenUnconnected=off
  wires:
  Signal1/1 -> Data_Sorter_Switch/3, Data_Sorter_Switch/1, Relational Operator2/1
  Relational Operator2/1 -> Data_Sorter_Switch1/2, Data_Sorter_Switch/2
  Signal2/1 -> Data_Sorter_Switch1/1, Data_Sorter_Switch1/3, Relational Operator2/2
  Data_Sorter_Switch1/1 -> Delay2/1
  Delay2/1 -> Low_Data/1
  Data_Sorter_Switch/1 -> Delay1/1
  Delay1/1 -> High_Data/1

== system Absolute_Block_Testing/Threshold_Estimator/Median2/Data_Sorter14 ==
  Signal1 : Inport  OutDataTypeStr=fixdt(1,16,12)  SampleTime=0.000022675736
  Signal2 : Inport  Port=2  OutDataTypeStr=fixdt(1,16,12)  SampleTime=0.000022675736
  Data_Sorter_Switch : Switch  OutDataTypeStr=fixdt(1,16,12)
  Data_Sorter_Switch1 : Switch  Threshold=1  OutDataTypeStr=fixdt(1,16,12)
  Delay1 : Delay  DelayLength=1  SampleTime=0.000022675736
  Delay2 : Delay  DelayLength=1  SampleTime=0.000022675736
  Relational Operator2 : RelationalOperator  Operator=<  OutDataTypeStr=fixdt(1,16,12)  RndMeth=Simplest
  High_Data : Outport  OutDataTypeStr=fixdt(1,16,12)  SampleTime=0.000022675736  VectorParamsAs1DForOutWhenUnconnected=off
  Low_Data : Outport  Port=2  OutDataTypeStr=fixdt(1,16,12)  SampleTime=0.000022675736  VectorParamsAs1DForOutWhenUnconnected=off
  wires:
  Signal1/1 -> Data_Sorter_Switch/3, Data_Sorter_Switch/1, Relational Operator2/1
  Relational Operator2/1 -> Data_Sorter_Switch1/2, Data_Sorter_Switch/2
  Signal2/1 -> Data_Sorter_Switch1/1, Data_Sorter_Switch1/3, Relational Operator2/2
  Data_Sorter_Switch1/1 -> Delay2/1
  Delay2/1 -> Low_Data/1
  Data_Sorter_Switch/1 -> Delay1/1
  Delay1/1 -> High_Data/1

== system Absolute_Block_Testing/Threshold_Estimator/Median2/Data_Sorter15 ==
  Signal1 : Inport  OutDataTypeStr=fixdt(1,16,12)  SampleTime=0.000022675736
  Signal2 : Inport  Port=2  OutDataTypeStr=fixdt(1,16,12)  SampleTime=0.000022675736
  Data_Sorter_Switch : Switch  OutDataTypeStr=fixdt(1,16,12)
  Data_Sorter_Switch1 : Switch  Threshold=1  OutDataTypeStr=fixdt(1,16,12)
  Delay1 : Delay  DelayLength=1  SampleTime=0.000022675736
  Delay2 : Delay  DelayLength=1  SampleTime=0.000022675736
  Relational Operator2 : RelationalOperator  Operator=<  OutDataTypeStr=fixdt(1,16,12)  RndMeth=Simplest
  High_Data : Outport  OutDataTypeStr=fixdt(1,16,12)  SampleTime=0.000022675736  VectorParamsAs1DForOutWhenUnconnected=off
  Low_Data : Outport  Port=2  OutDataTypeStr=fixdt(1,16,12)  SampleTime=0.000022675736  VectorParamsAs1DForOutWhenUnconnected=off
  wires:
  Signal1/1 -> Data_Sorter_Switch/3, Data_Sorter_Switch/1, Relational Operator2/1
  Relational Operator2/1 -> Data_Sorter_Switch1/2, Data_Sorter_Switch/2
  Signal2/1 -> Data_Sorter_Switch1/1, Data_Sorter_Switch1/3, Relational Operator2/2
  Data_Sorter_Switch1/1 -> Delay2/1
  Delay2/1 -> Low_Data/1
  Data_Sorter_Switch/1 -> Delay1/1
  Delay1/1 -> High_Data/1

== system Absolute_Block_Testing/Threshold_Estimator/Median2/Data_Sorter16 ==
  Signal1 : Inport  OutDataTypeStr=fixdt(1,16,12)  SampleTime=0.000022675736
  Signal2 : Inport  Port=2  OutDataTypeStr=fixdt(1,16,12)  SampleTime=0.000022675736
  Data_Sorter_Switch : Switch  OutDataTypeStr=fixdt(1,16,12)
  Delay1 : Delay  DelayLength=1  SampleTime=0.000022675736
  Relational Operator2 : RelationalOperator  Operator=<  OutDataTypeStr=fixdt(1,16,12)  RndMeth=Simplest
  High_Data : Outport  OutDataTypeStr=fixdt(1,16,12)  SampleTime=0.000022675736  VectorParamsAs1DForOutWhenUnconnected=off
  wires:
  Signal1/1 -> Data_Sorter_Switch/3, Data_Sorter_Switch/1, Relational Operator2/1
  Relational Operator2/1 -> Data_Sorter_Switch/2
  Signal2/1 -> Relational Operator2/2
  Data_Sorter_Switch/1 -> Delay1/1
  Delay1/1 -> High_Data/1

== system Absolute_Block_Testing/Threshold_Estimator/Median2/Data_Sorter17 ==
  Signal1 : Inport  OutDataTypeStr=fixdt(1,16,12)  SampleTime=0.000022675736
  Signal2 : Inport  Port=2  OutDataTypeStr=fixdt(1,16,12)  SampleTime=0.000022675736
  Data_Sorter_Switch1 : Switch  Threshold=1  OutDataTypeStr=fixdt(1,16,12)
  Delay2 : Delay  DelayLength=1  SampleTime=0.000022675736
  Relational Operator2 : RelationalOperator  Operator=<  OutDataTypeStr=fixdt(1,16,12)  RndMeth=Simplest
  Low_Data : Outport  OutDataTypeStr=fixdt(1,16,12)  SampleTime=0.000022675736  VectorParamsAs1DForOutWhenUnconnected=off
  wires:
  Signal1/1 -> Relational Operator2/1
  Relational Operator2/1 -> Data_Sorter_Switch1/2
  Signal2/1 -> Data_Sorter_Switch1/1, Data_Sorter_Switch1/3, Relational Operator2/2
  Data_Sorter_Switch1/1 -> Delay2/1
  Delay2/1 -> Low_Data/1

== system Absolute_Block_Testing/Threshold_Estimator/Median2/Data_Sorter18 ==
  Signal1 : Inport  OutDataTypeStr=fixdt(1,16,12)  SampleTime=0.000022675736
  Signal2 : Inport  Port=2  OutDataTypeStr=fixdt(1,16,12)  SampleTime=0.000022675736
  Data_Sorter_Switch : Switch  OutDataTypeStr=fixdt(1,16,12)
  Data_Sorter_Switch1 : Switch  Threshold=1  OutDataTypeStr=fixdt(1,16,12)
  Delay1 : Delay  DelayLength=1  SampleTime=0.000022675736
  Delay2 : Delay  DelayLength=1  SampleTime=0.000022675736
  Relational Operator2 : RelationalOperator  Operator=<  OutDataTypeStr=fixdt(1,16,12)  RndMeth=Simplest
  High_Data : Outport  OutDataTypeStr=fixdt(1,16,12)  SampleTime=0.000022675736  VectorParamsAs1DForOutWhenUnconnected=off
  Low_Data : Outport  Port=2  OutDataTypeStr=fixdt(1,16,12)  SampleTime=0.000022675736  VectorParamsAs1DForOutWhenUnconnected=off
  wires:
  Signal1/1 -> Data_Sorter_Switch/3, Data_Sorter_Switch/1, Relational Operator2/1
  Relational Operator2/1 -> Data_Sorter_Switch1/2, Data_Sorter_Switch/2
  Signal2/1 -> Data_Sorter_Switch1/1, Data_Sorter_Switch1/3, Relational Operator2/2
  Data_Sorter_Switch1/1 -> Delay2/1
  Delay2/1 -> Low_Data/1
  Data_Sorter_Switch/1 -> Delay1/1
  Delay1/1 -> High_Data/1

== system Absolute_Block_Testing/Threshold_Estimator/Median2/Data_Sorter19 ==
  Signal1 : Inport  OutDataTypeStr=fixdt(1,16,12)  SampleTime=0.000022675736
  Signal2 : Inport  Port=2  OutDataTypeStr=fixdt(1,16,12)  SampleTime=0.000022675736
  Data_Sorter_Switch : Switch  OutDataTypeStr=fixdt(1,16,12)
  Data_Sorter_Switch1 : Switch  Threshold=1  OutDataTypeStr=fixdt(1,16,12)
  Delay1 : Delay  DelayLength=1  SampleTime=0.000022675736
  Delay2 : Delay  DelayLength=1  SampleTime=0.000022675736
  Relational Operator2 : RelationalOperator  Operator=<  OutDataTypeStr=fixdt(1,16,12)  RndMeth=Simplest
  High_Data : Outport  OutDataTypeStr=fixdt(1,16,12)  SampleTime=0.000022675736  VectorParamsAs1DForOutWhenUnconnected=off
  Low_Data : Outport  Port=2  OutDataTypeStr=fixdt(1,16,12)  SampleTime=0.000022675736  VectorParamsAs1DForOutWhenUnconnected=off
  wires:
  Signal1/1 -> Data_Sorter_Switch/3, Data_Sorter_Switch/1, Relational Operator2/1
  Relational Operator2/1 -> Data_Sorter_Switch1/2, Data_Sorter_Switch/2
  Signal2/1 -> Data_Sorter_Switch1/1, Data_Sorter_Switch1/3, Relational Operator2/2
  Data_Sorter_Switch1/1 -> Delay2/1
  Delay2/1 -> Low_Data/1
  Data_Sorter_Switch/1 -> Delay1/1
  Delay1/1 -> High_Data/1

== system Absolute_Block_Testing/Threshold_Estimator/Median2/Data_Sorter2 ==
  Signal1 : Inport  OutDataTypeStr=fixdt(1,16,12)  SampleTime=0.000022675736
  Signal2 : Inport  Port=2  OutDataTypeStr=fixdt(1,16,12)  SampleTime=0.000022675736
  Data_Sorter_Switch : Switch  OutDataTypeStr=fixdt(1,16,12)
  Data_Sorter_Switch1 : Switch  Threshold=1  OutDataTypeStr=fixdt(1,16,12)
  Delay1 : Delay  DelayLength=1  SampleTime=0.000022675736
  Delay2 : Delay  DelayLength=1  SampleTime=0.000022675736
  Relational Operator2 : RelationalOperator  Operator=<  OutDataTypeStr=fixdt(1,16,12)  RndMeth=Simplest
  High_Data : Outport  OutDataTypeStr=fixdt(1,16,12)  SampleTime=0.000022675736  VectorParamsAs1DForOutWhenUnconnected=off
  Low_Data : Outport  Port=2  OutDataTypeStr=fixdt(1,16,12)  SampleTime=0.000022675736  VectorParamsAs1DForOutWhenUnconnected=off
  wires:
  Signal1/1 -> Data_Sorter_Switch/3, Data_Sorter_Switch/1, Relational Operator2/1
  Relational Operator2/1 -> Data_Sorter_Switch1/2, Data_Sorter_Switch/2
  Signal2/1 -> Data_Sorter_Switch1/1, Data_Sorter_Switch1/3, Relational Operator2/2
  Data_Sorter_Switch1/1 -> Delay2/1
  Delay2/1 -> Low_Data/1
  Data_Sorter_Switch/1 -> Delay1/1
  Delay1/1 -> High_Data/1

== system Absolute_Block_Testing/Threshold_Estimator/Median2/Data_Sorter20 ==
  Signal1 : Inport  OutDataTypeStr=fixdt(1,16,12)  SampleTime=0.000022675736
  Signal2 : Inport  Port=2  OutDataTypeStr=fixdt(1,16,12)  SampleTime=0.000022675736
  Data_Sorter_Switch1 : Switch  Threshold=1  OutDataTypeStr=fixdt(1,16,12)
  Delay2 : Delay  DelayLength=1  SampleTime=0.000022675736
  Relational Operator2 : RelationalOperator  Operator=<  OutDataTypeStr=fixdt(1,16,12)  RndMeth=Simplest
  Low_Data : Outport  OutDataTypeStr=fixdt(1,16,12)  SampleTime=0.000022675736  VectorParamsAs1DForOutWhenUnconnected=off
  wires:
  Signal1/1 -> Relational Operator2/1
  Relational Operator2/1 -> Data_Sorter_Switch1/2
  Signal2/1 -> Data_Sorter_Switch1/1, Data_Sorter_Switch1/3, Relational Operator2/2
  Data_Sorter_Switch1/1 -> Delay2/1
  Delay2/1 -> Low_Data/1

== system Absolute_Block_Testing/Threshold_Estimator/Median2/Data_Sorter21 ==
  Signal1 : Inport  OutDataTypeStr=fixdt(1,16,12)  SampleTime=0.000022675736
  Signal2 : Inport  Port=2  OutDataTypeStr=fixdt(1,16,12)  SampleTime=0.000022675736
  Data_Sorter_Switch : Switch  OutDataTypeStr=fixdt(1,16,12)
  Delay1 : Delay  DelayLength=1  SampleTime=0.000022675736
  Relational Operator2 : RelationalOperator  Operator=<  OutDataTypeStr=fixdt(1,16,12)  RndMeth=Simplest
  High_Data : Outport  OutDataTypeStr=fixdt(1,16,12)  SampleTime=0.000022675736  VectorParamsAs1DForOutWhenUnconnected=off
  wires:
  Signal1/1 -> Data_Sorter_Switch/3, Data_Sorter_Switch/1, Relational Operator2/1
  Relational Operator2/1 -> Data_Sorter_Switch/2
  Signal2/1 -> Relational Operator2/2
  Data_Sorter_Switch/1 -> Delay1/1
  Delay1/1 -> High_Data/1

== system Absolute_Block_Testing/Threshold_Estimator/Median2/Data_Sorter22 ==
  Signal1 : Inport  OutDataTypeStr=fixdt(1,16,12)  SampleTime=0.000022675736
  Signal2 : Inport  Port=2  OutDataTypeStr=fixdt(1,16,12)  SampleTime=0.000022675736
  Data_Sorter_Switch1 : Switch  Threshold=1  OutDataTypeStr=fixdt(1,16,12)
  Delay2 : Delay  DelayLength=1  SampleTime=0.000022675736
  Relational Operator2 : RelationalOperator  Operator=<  OutDataTypeStr=fixdt(1,16,12)  RndMeth=Simplest
  Low_Data : Outport  OutDataTypeStr=fixdt(1,16,12)  SampleTime=0.000022675736  VectorParamsAs1DForOutWhenUnconnected=off
  wires:
  Signal1/1 -> Relational Operator2/1
  Relational Operator2/1 -> Data_Sorter_Switch1/2
  Signal2/1 -> Data_Sorter_Switch1/1, Data_Sorter_Switch1/3, Relational Operator2/2
  Data_Sorter_Switch1/1 -> Delay2/1
  Delay2/1 -> Low_Data/1

== system Absolute_Block_Testing/Threshold_Estimator/Median2/Data_Sorter23 ==
  Signal1 : Inport  OutDataTypeStr=fixdt(1,16,12)  SampleTime=0.000022675736
  Signal2 : Inport  Port=2  OutDataTypeStr=fixdt(1,16,12)  SampleTime=0.000022675736
  Data_Sorter_Switch : Switch  OutDataTypeStr=fixdt(1,16,12)
  Delay1 : Delay  DelayLength=1  SampleTime=0.000022675736
  Relational Operator2 : RelationalOperator  Operator=<  OutDataTypeStr=fixdt(1,16,12)  RndMeth=Simplest
  High_Data : Outport  OutDataTypeStr=fixdt(1,16,12)  SampleTime=0.000022675736  VectorParamsAs1DForOutWhenUnconnected=off
  wires:
  Signal1/1 -> Data_Sorter_Switch/3, Data_Sorter_Switch/1, Relational Operator2/1
  Relational Operator2/1 -> Data_Sorter_Switch/2
  Signal2/1 -> Relational Operator2/2
  Data_Sorter_Switch/1 -> Delay1/1
  Delay1/1 -> High_Data/1

== system Absolute_Block_Testing/Threshold_Estimator/Median2/Data_Sorter24 ==
  Signal1 : Inport  OutDataTypeStr=fixdt(1,16,12)  SampleTime=0.000022675736
  Signal2 : Inport  Port=2  OutDataTypeStr=fixdt(1,16,12)  SampleTime=0.000022675736
  Data_Sorter_Switch : Switch  OutDataTypeStr=fixdt(1,16,12)
  Data_Sorter_Switch1 : Switch  Threshold=1  OutDataTypeStr=fixdt(1,16,12)
  Delay1 : Delay  DelayLength=1  SampleTime=0.000022675736
  Delay2 : Delay  DelayLength=1  SampleTime=0.000022675736
  Relational Operator2 : RelationalOperator  Operator=<  OutDataTypeStr=fixdt(1,16,12)  RndMeth=Simplest
  High_Data : Outport  OutDataTypeStr=fixdt(1,16,12)  SampleTime=0.000022675736  VectorParamsAs1DForOutWhenUnconnected=off
  Low_Data : Outport  Port=2  OutDataTypeStr=fixdt(1,16,12)  SampleTime=0.000022675736  VectorParamsAs1DForOutWhenUnconnected=off
  wires:
  Signal1/1 -> Data_Sorter_Switch/3, Data_Sorter_Switch/1, Relational Operator2/1
  Relational Operator2/1 -> Data_Sorter_Switch1/2, Data_Sorter_Switch/2
  Signal2/1 -> Data_Sorter_Switch1/1, Data_Sorter_Switch1/3, Relational Operator2/2
  Data_Sorter_Switch1/1 -> Delay2/1
  Delay2/1 -> Low_Data/1
  Data_Sorter_Switch/1 -> Delay1/1
  Delay1/1 -> High_Data/1

== system Absolute_Block_Testing/Threshold_Estimator/Median2/Data_Sorter3 ==
  Signal1 : Inport  OutDataTypeStr=fixdt(1,16,12)  SampleTime=0.000022675736
  Signal2 : Inport  Port=2  OutDataTypeStr=fixdt(1,16,12)  SampleTime=0.000022675736
  Data_Sorter_Switch : Switch  OutDataTypeStr=fixdt(1,16,12)
  Data_Sorter_Switch1 : Switch  Threshold=1  OutDataTypeStr=fixdt(1,16,12)
  Delay1 : Delay  DelayLength=1  SampleTime=0.000022675736
  Delay2 : Delay  DelayLength=1  SampleTime=0.000022675736
  Relational Operator2 : RelationalOperator  Operator=<  OutDataTypeStr=fixdt(1,16,12)  RndMeth=Simplest
  High_Data : Outport  OutDataTypeStr=fixdt(1,16,12)  SampleTime=0.000022675736  VectorParamsAs1DForOutWhenUnconnected=off
  Low_Data : Outport  Port=2  OutDataTypeStr=fixdt(1,16,12)  SampleTime=0.000022675736  VectorParamsAs1DForOutWhenUnconnected=off
  wires:
  Signal1/1 -> Data_Sorter_Switch/3, Data_Sorter_Switch/1, Relational Operator2/1
  Relational Operator2/1 -> Data_Sorter_Switch1/2, Data_Sorter_Switch/2
  Signal2/1 -> Data_Sorter_Switch1/1, Data_Sorter_Switch1/3, Relational Operator2/2
  Data_Sorter_Switch1/1 -> Delay2/1
  Delay2/1 -> Low_Data/1
  Data_Sorter_Switch/1 -> Delay1/1
  Delay1/1 -> High_Data/1

== system Absolute_Block_Testing/Threshold_Estimator/Median2/Data_Sorter4 ==
  Signal1 : Inport  OutDataTypeStr=fixdt(1,16,12)  SampleTime=0.000022675736
  Signal2 : Inport  Port=2  OutDataTypeStr=fixdt(1,16,12)  SampleTime=0.000022675736
  Data_Sorter_Switch : Switch  OutDataTypeStr=fixdt(1,16,12)
  Data_Sorter_Switch1 : Switch  Threshold=1  OutDataTypeStr=fixdt(1,16,12)
  Delay1 : Delay  DelayLength=1  SampleTime=0.000022675736
  Delay2 : Delay  DelayLength=1  SampleTime=0.000022675736
  Relational Operator2 : RelationalOperator  Operator=<  OutDataTypeStr=fixdt(1,16,12)  RndMeth=Simplest
  High_Data : Outport  OutDataTypeStr=fixdt(1,16,12)  SampleTime=0.000022675736  VectorParamsAs1DForOutWhenUnconnected=off
  Low_Data : Outport  Port=2  OutDataTypeStr=fixdt(1,16,12)  SampleTime=0.000022675736  VectorParamsAs1DForOutWhenUnconnected=off
  wires:
  Signal1/1 -> Data_Sorter_Switch/3, Data_Sorter_Switch/1, Relational Operator2/1
  Relational Operator2/1 -> Data_Sorter_Switch1/2, Data_Sorter_Switch/2
  Signal2/1 -> Data_Sorter_Switch1/1, Data_Sorter_Switch1/3, Relational Operator2/2
  Data_Sorter_Switch1/1 -> Delay2/1
  Delay2/1 -> Low_Data/1
  Data_Sorter_Switch/1 -> Delay1/1
  Delay1/1 -> High_Data/1

== system Absolute_Block_Testing/Threshold_Estimator/Median2/Data_Sorter5 ==
  Signal1 : Inport  OutDataTypeStr=fixdt(1,16,12)  SampleTime=0.000022675736
  Signal2 : Inport  Port=2  OutDataTypeStr=fixdt(1,16,12)  SampleTime=0.000022675736
  Data_Sorter_Switch : Switch  OutDataTypeStr=fixdt(1,16,12)
  Data_Sorter_Switch1 : Switch  Threshold=1  OutDataTypeStr=fixdt(1,16,12)
  Delay1 : Delay  DelayLength=1  SampleTime=0.000022675736
  Delay2 : Delay  DelayLength=1  SampleTime=0.000022675736
  Relational Operator2 : RelationalOperator  Operator=<  OutDataTypeStr=fixdt(1,16,12)  RndMeth=Simplest
  High_Data : Outport  OutDataTypeStr=fixdt(1,16,12)  SampleTime=0.000022675736  VectorParamsAs1DForOutWhenUnconnected=off
  Low_Data : Outport  Port=2  OutDataTypeStr=fixdt(1,16,12)  SampleTime=0.000022675736  VectorParamsAs1DForOutWhenUnconnected=off
  wires:
  Signal1/1 -> Data_Sorter_Switch/3, Data_Sorter_Switch/1, Relational Operator2/1
  Relational Operator2/1 -> Data_Sorter_Switch1/2, Data_Sorter_Switch/2
  Signal2/1 -> Data_Sorter_Switch1/1, Data_Sorter_Switch1/3, Relational Operator2/2
  Data_Sorter_Switch1/1 -> Delay2/1
  Delay2/1 -> Low_Data/1
  Data_Sorter_Switch/1 -> Delay1/1
  Delay1/1 -> High_Data/1

== system Absolute_Block_Testing/Threshold_Estimator/Median2/Data_Sorter6 ==
  Signal1 : Inport  OutDataTypeStr=fixdt(1,16,12)  SampleTime=0.000022675736
  Signal2 : Inport  Port=2  OutDataTypeStr=fixdt(1,16,12)  SampleTime=0.000022675736
  Data_Sorter_Switch : Switch  OutDataTypeStr=fixdt(1,16,12)
  Data_Sorter_Switch1 : Switch  Threshold=1  OutDataTypeStr=fixdt(1,16,12)
  Delay1 : Delay  DelayLength=1  SampleTime=0.000022675736
  Delay2 : Delay  DelayLength=1  SampleTime=0.000022675736
  Relational Operator2 : RelationalOperator  Operator=<  OutDataTypeStr=fixdt(1,16,12)  RndMeth=Simplest
  High_Data : Outport  OutDataTypeStr=fixdt(1,16,12)  SampleTime=0.000022675736  VectorParamsAs1DForOutWhenUnconnected=off
  Low_Data : Outport  Port=2  OutDataTypeStr=fixdt(1,16,12)  SampleTime=0.000022675736  VectorParamsAs1DForOutWhenUnconnected=off
  wires:
  Signal1/1 -> Data_Sorter_Switch/3, Data_Sorter_Switch/1, Relational Operator2/1
  Relational Operator2/1 -> Data_Sorter_Switch1/2, Data_Sorter_Switch/2
  Signal2/1 -> Data_Sorter_Switch1/1, Data_Sorter_Switch1/3, Relational Operator2/2
  Data_Sorter_Switch1/1 -> Delay2/1
  Delay2/1 -> Low_Data/1
  Data_Sorter_Switch/1 -> Delay1/1
  Delay1/1 -> High_Data/1

== system Absolute_Block_Testing/Threshold_Estimator/Median2/Data_Sorter7 ==
  Signal1 : Inport  OutDataTypeStr=fixdt(1,16,12)  SampleTime=0.000022675736
  Signal2 : Inport  Port=2  OutDataTypeStr=fixdt(1,16,12)  SampleTime=0.000022675736
  Data_Sorter_Switch : Switch  OutDataTypeStr=fixdt(1,16,12)
  Data_Sorter_Switch1 : Switch  Threshold=1  OutDataTypeStr=fixdt(1,16,12)
  Delay1 : Delay  DelayLength=1  SampleTime=0.000022675736
  Delay2 : Delay  DelayLength=1  SampleTime=0.000022675736
  Relational Operator2 : RelationalOperator  Operator=<  OutDataTypeStr=fixdt(1,16,12)  RndMeth=Simplest
  High_Data : Outport  OutDataTypeStr=fixdt(1,16,12)  SampleTime=0.000022675736  VectorParamsAs1DForOutWhenUnconnected=off
  Low_Data : Outport  Port=2  OutDataTypeStr=fixdt(1,16,12)  SampleTime=0.000022675736  VectorParamsAs1DForOutWhenUnconnected=off
  wires:
  Signal1/1 -> Data_Sorter_Switch/3, Data_Sorter_Switch/1, Relational Operator2/1
  Relational Operator2/1 -> Data_Sorter_Switch1/2, Data_Sorter_Switch/2
  Signal2/1 -> Data_Sorter_Switch1/1, Data_Sorter_Switch1/3, Relational Operator2/2
  Data_Sorter_Switch1/1 -> Delay2/1
  Delay2/1 -> Low_Data/1
  Data_Sorter_Switch/1 -> Delay1/1
  Delay1/1 -> High_Data/1
